simulink model "task2_test"  (R2021a)
settings: Solver=VariableStepAuto  StartTime=0.0  StopTime=10.0  RelTol=1e-3
values from neighbouring files (symbols this model uses):
  T_l = T_l_range(1,i)    [Task1.m]    (also in Task2.m = 0.52; Task2b.m; Task3.m; Task4.m = T_l_range(1,k))
undefined symbols (not defined in the file or in its folder): tf1
settings Model: Creator=Usamat980  LastModifiedBy=Usamat980

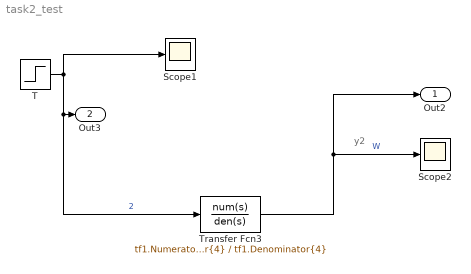
== system task2_test ==
  note: y2
  Scope1 : Scope
  Scope2 : Scope
  T : Step  Time=0  After=T_l  SampleTime=0
  Transfer Fcn3 : TransferFcn  Numerator=tf1.Numerator{4}  Denominator=tf1.Denominator{4}
  Out2 : Outport
  Out3 : Outport  Port=2
  wires:
  T/1 -> Out3/1, Transfer Fcn3/1, Scope1/1  "2"
  Transfer Fcn3/1 -> Scope2/1, Out2/1  "W"
